simulink model "analog_adapt"  (R2020b)
settings: Solver=VariableStepAuto  StartTime=0.0  StopTime=20  RelTol=1e-3
libraries: dsparch4 x1, simulink x1, dspadpt3 x1
settings Model: Creator=shiva  LastModifiedBy=shiva

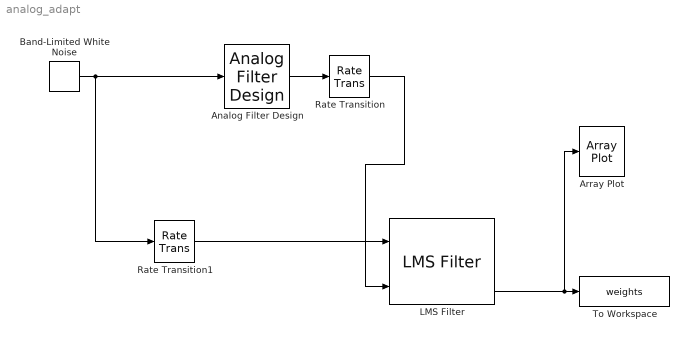
== system analog_adapt ==
  Analog Filter Design : dsparch4/Analog Filter Design  method=Butterworth  filttype=Lowpass  N=8  Wlo=12560  Whi=80  Rp=2  Rs=40
  Array Plot : ArrayPlot
  Band-Limited White Noise : simulink/Sources/Band-Limited White Noise  Cov=[1]  Ts=125*10^-6  seed=[23341]
  LMS Filter : dspadpt3/LMS Filter  Algo=Normalized LMS  L=99  stepflag=Dialog  mu=0.01  leakage=1.0  ic=0  Adapt=off  resetflag=None  weights=on  addnparflag=off  roundingMode=Floor  overflowMode=off
      settings: SourceProductBaseCode=DS
  Rate Transition : RateTransition  OutPortSampleTime=125*10^-6
  Rate Transition1 : RateTransition  OutPortSampleTime=125*10^-6
  To Workspace : ToWorkspace  VariableName=weights  SaveFormat=Timeseries  SampleTime=-1
      settings: MaxDataPoints=1
  wires:
  Band-Limited White Noise/1 -> Rate Transition1/1, Analog Filter Design/1
  Analog Filter Design/1 -> Rate Transition/1
  Rate Transition/1 -> LMS Filter/2
  Rate Transition1/1 -> LMS Filter/1
  LMS Filter/3 -> Array Plot/1, To Workspace/1
